simulink model "MainModel_Working_version_With_AAIR"  (R2020a)
settings: Solver=FixedStepAuto  StartTime=0.0  StopTime=10  FixedStep=1e-3  RelTol=1e-3  EnableMultiTasking=on
undefined symbols (not defined in the file): A0, A3, D0, D1, D10, D11, D12, D13, D2, D3, D4, D5, D6, D7, D8, D9, PTA0, PTA1, PTA2, PTB11, PTB2, PTB23, PTB9, PTC16, PTC17, PTC2, PTC3, PTC4, PTD0, PTD1, PTD2, PTD3
libraries: frdmk64flib x19
(part 2 of 2)

== stateflow chart MainModel_Working_version_With_AAIR/1.1.2 InputProcessing/1.1.2.1 PulsePeriodDetermination ==
  state default
    entry:
  state UnsensedModes
    entry:
    HR_Ready = true
    exit:
    HR_Ready = false
  state AtrialRateDetection
    state default
      entry:
      pulse_finished = false
      time_between_pulses = 0
    state setARPasDeltaT
      entry:
      time_between_pulses = ARP
    state awaitNewPulse
      entry:
      time_between_pulses = time_between_pulses+1
    state newPulseDetected
      entry:
      pulse_finished = true
      HR_Ready = true
    state resetDeltaT
      entry:
      pulse_finished = false
      time_between_pulses = ARP
    (default) -> AtrialRateDetection.default
    AtrialRateDetection.default -> setARPasDeltaT : [AtrialPulseDetected == 1]
    setARPasDeltaT -> (junction 59) : [after(ARP,msec)]
    AtrialRateDetection.awaitNewPulse -> AtrialRateDetection.awaitNewPulse [order 1] : [AtrialPulseDetected == 0]
    (junction 59) -> AtrialRateDetection.awaitNewPulse [order 1] : [AtrialPulseDetected ==0]
    (junction 59) -> AtrialRateDetection.newPulseDetected [order 2] : [AtrialPulseDetected == 1]
    AtrialRateDetection.resetDeltaT -> (junction 59) : [after(ARP-1,msec)]
    AtrialRateDetection.awaitNewPulse -> AtrialRateDetection.newPulseDetected [order 2] : [AtrialPulseDetected == 1]
    AtrialRateDetection.newPulseDetected -> AtrialRateDetection.resetDeltaT : [after(1,msec)]
  state VenticularRateDetection
    state default
      entry:
      pulse_finished = false
      time_between_pulses = 0
    state setVRPasDeltaT
      entry:
      time_between_pulses = VRP
    state awaitNewPulse
      entry:
      time_between_pulses = time_between_pulses+1
    state newPulseDetected
      entry:
      pulse_finished = true
      HR_Ready = true
    state resetDeltaT
      entry:
      pulse_finished = false
      time_between_pulses = VRP
    (default) -> VenticularRateDetection.default
    VenticularRateDetection.default -> setVRPasDeltaT : [VentricularPulseDetected == 1]
    setVRPasDeltaT -> (junction 93) : [after(VRP,msec)]
    VenticularRateDetection.awaitNewPulse -> VenticularRateDetection.awaitNewPulse [order 1] : [VentricularPulseDetected == 0]
    (junction 93) -> VenticularRateDetection.awaitNewPulse [order 1] : [VentricularPulseDetected ==0]
    (junction 93) -> VenticularRateDetection.newPulseDetected [order 2] : [VentricularPulseDetected == 1]
    VenticularRateDetection.resetDeltaT -> (junction 93) : [after(VRP-1,msec)]
    VenticularRateDetection.awaitNewPulse -> VenticularRateDetection.newPulseDetected [order 2] : [VentricularPulseDetected == 1]
    VenticularRateDetection.newPulseDetected -> VenticularRateDetection.resetDeltaT : [after(1,msec)]
  (default) -> default
  default -> UnsensedModes [order 2] : [Mode == 100 || Mode == 200]
  UnsensedModes -> default : [Mode ~= 100 && Mode ~= 200]
  default -> AtrialRateDetection [order 1] : [Mode == 112]
  AtrialRateDetection -> default : [Mode ~= 112]
  default -> VenticularRateDetection [order 3] : [Mode == 222]
  VenticularRateDetection -> default : [Mode ~= 222]
  data: Mode input; time_between_pulses output uint32; pulse_finished output boolean; AtrialPulseDetected input boolean; VentricularPulseDetected input boolean; VRP input uint32; ARP input uint32; HR_Ready output boolean

== stateflow chart MainModel_Working_version_With_AAIR/1.1.1 HardwareInputMapping/HeartChamberPulseDetection ==
  state default
    entry:
    LED_STATE = false
  state led_on
    entry:
    LED_STATE = true
  (default) -> default
  default -> led_on : [in_voltage ==1]
  led_on -> default : [in_voltage ~= 1]
  data: LED_STATE output boolean; in_voltage input

== stateflow chart MainModel_Working_version_With_AAIR/1.1.2 InputProcessing/1.1.2.4 CalculateUnsensedPace/Chart ==
  state init
    entry:
  state Activity_Greater_than_Threshold
    entry:
    u1 = LowerRateLimit + ResponseFactor*(activity_magnitude - AThresh)/(sqrt(48)-AThresh)*(MSR-LowerRateLimit);
  state Activity_Less_than_Threshold
    entry:
    f_aoorInterval = 1/(LowerRateLimit/60000);
  state MSR_greater_than_u1
    entry:
    XXIR_ppm = u1;
    f_aoorInterval = 1/(u1/60000);
  state MSR_less_than_u1
    entry:
    XXIR_ppm = MSR;
    f_aoorInterval = 1/(MSR/60000);
  MSR_greater_than_u1 -> init : [[after(1,msec) ]]
  (default) -> init
  Activity_Less_than_Threshold -> init : [after(1,msec) ]
  MSR_less_than_u1 -> init : [[after(1,msec) ] ]
  init -> Activity_Greater_than_Threshold [order 1] : [activity_magnitude > AThresh]
  init -> Activity_Less_than_Threshold [order 2] : [activity_magnitude <= AThresh]
  Activity_Greater_than_Threshold -> MSR_greater_than_u1 [order 1] : [MSR > u1]
  Activity_Greater_than_Threshold -> MSR_less_than_u1 [order 2] : [MSR <= u1]
  data: XXIR_ppm output uint32; AThresh input; MSR input uint32; LowerRateLimit input; ResponseFactor input; activity_magnitude input; f_aoorInterval output uint32; u1 local

== stateflow chart MainModel_Working_version_With_AAIR/1.1.1 HardwareInputMapping/Chart ==
  state Safety_Check
    entry:
    if Mode_U == 1000 || Mode_U == 2000 || Mode_U == 110
    Mode = Mode_U;
    end
    if  50<upper_rate_limit_U<175
    upper_rate_limit = upper_rate_limit_U;
    end
    if  50<lower_rate_limit_U<100
    lower_rate_limit = lower_rate_limit_U;
    end
  note: [[0,0,0,0,0,0,0,0],[1,1,1,1,1,1,1,1]]
  state Initial_State
    % Set default values for parameters
    entry:
    Mode = 100;
    upper_rate_limit = 175;
    lower_rate_limit = 50;
    atrial_amplitude = 3.75;
    atrial_pulse_width = 0.4;
    ventricular_amplitude = 3.75;
    ventricular_pulse_width = 1;
    a_r_p = 250;
    p_v_a_r_p = 250;
    h_r_l = 45;
    r_s_up = 0.09;
    r_s_down = 0.09;
    ventricular_sensitivity = 2.5;
    atrial_sensitivity = 2.75
    v_r_p = 320;
    hysterisis_flag = 0; % should talk about it
    activity_threshold = 2;
    ReactionTime = 1;
    ResponseFactor = 6;
    RecoveryTime = 1;
    MSR = 120;
  state Update_State
    entry:
    Mode_U = typecast(rx_data(3:6), 'uint32');
    upper_rate_limit_U  = typecast(rx_data(7:10), 'uint32');
    lower_rate_limit_U = typecast(rx_data(11:14), 'uint32');
    atrial_amplitude_U = typecast(rx_data(15:18), 'single');
    atrial_pulse_width_U = typecast(rx_data(19:26), 'double');
    ventricular_amplitude_U = typecast(rx_data(27:30), 'single');
    ventricular_pulse_width_U = typecast(rx_data(31:38), 'double');
    a_r_p_U = typecast(rx_data(39:42), 'uint32');
    p_v_a_r_p_U =typecast(rx_data(43:46), 'uint32');
    h_r_l_U= typecast(rx_data(47:50), 'uint32');
    r_s_up_U =typecast(rx_data(51:58), 'double');
    r_s_down_U = typecast(rx_data(59:66), 'double');
    atrial_sensitivity_U = typecast(rx_data(67:70), 'single');
    ventricular_sensitivity_U = typecast(rx_data(71:74), 'single');
    v_r_p_U = typecast(rx_data(75:78), 'uint32');
    activity_threshold_U = typecast(rx_data(79:82), 'uint32');
    ReactionTime_U = typecast(rx_data(83:86), 'uint32');
    ResponseFactor_U = typecast(rx_data(87:90), 'uint32');
    RecoveryTime_U = typecast(rx_data(91:94), 'uint32');
    MSR_U = typecast(rx_data(95:98), 'uint32');
    hysterisis_flag_U = typecast(rx_data(99), 'uint8');
  state Standby
  Safety_Check -> Standby
  (default) -> Initial_State
  Update_State -> Safety_Check
  (junction 12) -> Update_State : [[rx_data(2) == hex2dec('55')]]
  Initial_State -> Standby
  Standby -> (junction 7) : [status==[0]]
  (junction 7) -> (junction 12) : [[rx_data(1) == hex2dec('16')]]
  data: rx_data input; status input; MSR output; ReactionTime output; Mode output; RecoveryTime output; ResponseFactor output; a_r_p output; activity_threshold output; atrial_amplitude output; atrial_pulse_width output; atrial_sensitivity output; h_r_l output; hysterisis_flag output; lower_rate_limit output; p_v_a_r_p output; r_s_down output; r_s_up output; upper_rate_limit output; v_r_p output; ventricular_amplitude output; ventricular_pulse_width output; ventricular_sensitivity output; MSR_U local; Mode_U local; ReactionTime_U local; RecoveryTime_U local; ResponseFactor_U local; a_r_p_U local; activity_threshold_U local; atrial_amplitude_U local; atrial_pulse_width_U local; atrial_sensitivity_U local; h_r_l_U local; hysterisis_flag_U local; lower_rate_limit_U local; p_v_a_r_p_U local; r_s_down_U local; r_s_up_U local; upper_rate_limit_U local; v_r_p_U local; ventricular_amplitude_U local; ventricular_pulse_width_U local; ventricular_sensitivity_U local
